simulink library "lib_wheel2"  (Simulink 4.1.1)
values from neighbouring files (symbols this model uses):
  logFlag = 1    [advSACompMaskInit.m]    (also in advSACompMaskInitR13.m)
undefined symbols (not defined in the file or in its folder): lib_help, NOTES, veh_air_density, veh_CD, veh_cg_height, veh_FA, veh_front_wt_frac, veh_gravity, veh_roadwheel_radius, veh_rr_a, veh_rr_alpha, veh_rr_b, veh_rr_beta, veh_rr_c, veh_wheelbase, wh_1st_rrc, wh_2nd_rrc, wh_axle_loss_mass, wh_axle_loss_trq, wh_fa_dl_brake_frac, wh_fa_dl_brake_mph, wh_fa_fric_brake_frac, wh_fa_fric_brake_mph, wh_front_active_bool, wh_inertia, wh_max_front_brake_force, wh_max_rear_brake_force, wh_pressure, wh_radius, wh_rear_active_bool, wh_slip, wh_slip_force_coeff
libraries: lib_wheel2 x61, lib_vehicle x2, lib_etc x2, lib_controls x2, lib_wheel x1
(part 7 of 14)

== system lib_wheel2/Submodels/front and rear brake controller (achievable)/braking force supplied by front friction brakes (N)/Block NOTES ==
  note: The variable "wh_max_front_fric_brake_force_N" must be assigned a positive value.
  note: If all braking was intended to be done by the drivetrain, the front friction brakes will do 60% of the braking.
  note: where the denominator can also be expressed as [1 - front_axle_drivetrain_brake_fraction(vehicle speed)].
  note: [front_axle_friction_brake_fraction(vehicle speed)]
      | ------------------------------------------------------------------------------
      | [front_axle_friction_brake_fraction(vehicle speed) + rear_axle_friction_brake_fraction(vehicle speed)]
  note: If additional braking force is required to meet the specified deceleration, input #1 will be negative.
      | The fraction of the additional req'd braking force made up by the front-axle friction brakes is given by:

== system lib_wheel2/Submodels/traction control 2 axle/apply tire traction limit to req'd speed (m/s)/Block NOTES ==
  note: This block limits the requested speed by the maximum and minimum attainable given the maximum traction of the tires.
      | That is, acceleration and braking maneuvers are limited to the point of imminent skidding.
  note: The above equations are derived by solving F_maxaccel=mass*a_max for the maximum or minimum speed at the end of the time step,
      | given that F_maxaccel depends on the weight borne by the front tires which in turn depends on the vehicle's acceleration rate.
  note: Front-wheel drive is assumed, and weight transfer due to acceleration is included in the calculation of maximum tractive force.

== system lib_wheel2/Submodels/traction control 2 axle/apply tire traction limit to req'd speed (m/s)/max speed at END of time step given tire traction limit (m/s) ==
  in_1 : Inport  Port=1  LatchInput=off
  in_2 : Inport  Port=2  LatchInput=off
  Fcn : Fcn  Expr=1/u
  Product : Product  Inputs=2  Multiplication=Element-wise(.*)  SaturateOnIntegerOverflow=on
  out_1 : Outport  Port=1  InitialOutput=0
  wires:
  in_1/1 -> Product/1
  Fcn/1 -> Product/2
  Product/1 -> out_1/1
  in_2/1 -> Fcn/1

== system lib_wheel2/Submodels/traction control 2 axle/apply tire traction limit to req'd speed (m/s)/min speed at END of time step given tire traction limit (m/s) ==
  in_1 : Inport  Port=1  LatchInput=off
  in_2 : Inport  Port=2  LatchInput=off
  Fcn : Fcn  Expr=1/u
  Product : Product  Inputs=2  Multiplication=Element-wise(.*)  SaturateOnIntegerOverflow=on
  out_1 : Outport  Port=1  InitialOutput=0
  wires:
  in_2/1 -> Fcn/1
  Product/1 -> out_1/1
  Fcn/1 -> Product/2
  in_1/1 -> Product/1

== system lib_wheel2/Submodels/traction control 2 axle/apply tire traction limit to req'd speed (m/s)/rear slip terms ==
  initial speed : Inport  Port=1  LatchInput=off
  1/dt : Inport  Port=2  LatchInput=off
  sin(theta) : Inport  Port=3  LatchInput=off
  Constant12 : Constant  Value=max(wh_slip_force_coeff)*(-1*veh_cg_height)/veh_wheelbase
  Constant8 : Constant  Value=veh_gravity
  Product13 : Product  Inputs=3  Multiplication=Element-wise(.*)  SaturateOnIntegerOverflow=on
  Product14 : Product  Inputs=4  Multiplication=Element-wise(.*)  SaturateOnIntegerOverflow=on
  current veh mass : lib_wheel2/Submodels/current veh mass
      settings: RTWFcnNameOpts=Auto  RTWFileNameOpts=Auto
  Out1 : Outport  Port=1
  Out2 : Outport  Port=2
  wires:
  sin(theta)/1 -> Product13/3
  Product13/1 -> Out2/1
  1/dt/1 -> Product14/3
  Product14/1 -> Out1/1
  initial speed/1 -> Product14/2
  current veh mass/1 -> Product14/4
  Constant8/1 -> Product13/2
  Constant12/1 -> Product13/1, Product14/1

== system lib_wheel2/Submodels/traction control 2 axle/enforce max.  front axle tractive force  due to slip (N)/Block NOTES ==
  note: No more force will be requested of the drivetrain than can be transmitted by the front tires.
      | This transmittable force is computed taking into account the slip characteristics of the tires
      | and the variable, acceleration-dependent weight borne by the front axle.

== system lib_wheel2/Submodels/traction control 2 axle/enforce max.  front axle tractive force  due to slip (N)/front ==
  In1 : Inport  Port=1  LatchInput=off
  In2 : Inport  Port=2  LatchInput=off
  Clock : Clock
      settings: DisplayTime=off  Decimation=10
  Constant : Constant  Orientation=left  Value=veh_cg_height/veh_wheelbase
  Constant1 : Constant  Value=veh_gravity*veh_front_wt_frac
  Gain1 : Gain  Gain=2  Multiplication=Element-wise(K.*u)  SaturateOnIntegerOverflow=on
  Gain2 : Gain  Gain=veh_gravity  Multiplication=Element-wise(K.*u)  SaturateOnIntegerOverflow=on
  Memory1 : Memory  X0=-0.1  InheritSampleTime=off
      settings: RTWStateStorageClass=Auto
  Product : Product  Inputs=*/  Multiplication=Element-wise(.*)  SaturateOnIntegerOverflow=on
  Product1 : Product  Inputs=3  Multiplication=Element-wise(.*)  SaturateOnIntegerOverflow=on
  Product3 : Product  Inputs=3  Multiplication=Element-wise(.*)  SaturateOnIntegerOverflow=on
  Sum : Sum  Inputs=+-  SaturateOnIntegerOverflow=on
  Sum1 : Sum  Inputs=+-  SaturateOnIntegerOverflow=on
  Sum2 : Sum  Inputs=++  SaturateOnIntegerOverflow=on
  Trig Fn : Trigonometry  Operator=atan  OutputSignalType=auto
  Trig Fn1 : Trigonometry  Operator=sin  OutputSignalType=auto
  Trig Fn2 : Trigonometry  Operator=cos  OutputSignalType=auto
  current veh mass2 : lib_wheel2/Submodels/current veh mass
      settings: RTWFcnNameOpts=Auto  RTWFileNameOpts=Auto
  weight on front axle (N)1 : Sum  Inputs=-+  SaturateOnIntegerOverflow=on
  Out1 : Outport  Port=1
  wires:
  weight on front axle (N)1/1 -> Out1/1
  In2/1 -> Sum/2
  In1/1 -> Sum/1
  current veh mass2/1 -> Product3/1, Product1/3
  Trig Fn2/1 -> Product3/2
  Constant1/1 -> Product3/3
  Product3/1 -> weight on front axle (N)1/2
  Trig Fn/1 -> Trig Fn2/1, Trig Fn1/1
  Gain2/1 -> Sum2/2
  Trig Fn1/1 -> Gain2/1
  [grade] -> Trig Fn/1
  Sum2/1 -> Product1/2
  Gain1/1 -> Sum2/1
  Product/1 -> Gain1/1
  Sum1/1 -> Product/2
  Memory1/1 -> Sum1/2
  Clock/1 -> Memory1/1, Sum1/1
  Sum/1 -> Product/1
  Constant/1 -> Product1/1
  Product1/1 -> weight on front axle (N)1/1

== system lib_wheel2/Submodels/traction control 2 axle/enforce max.  front axle tractive force  due to slip (N)/rear ==
  In1 : Inport  Port=1  LatchInput=off
  In2 : Inport  Port=2  LatchInput=off
  Clock : Clock
      settings: DisplayTime=off  Decimation=10
  Constant : Constant  Orientation=left  Value=(-1*veh_cg_height)/veh_wheelbase
  Constant1 : Constant  Value=veh_gravity*(1-veh_front_wt_frac)
  Gain1 : Gain  Gain=2  Multiplication=Element-wise(K.*u)  SaturateOnIntegerOverflow=on
  Gain2 : Gain  Gain=veh_gravity  Multiplication=Element-wise(K.*u)  SaturateOnIntegerOverflow=on
  Memory1 : Memory  X0=-0.1  InheritSampleTime=off
      settings: RTWStateStorageClass=Auto
  Product : Product  Inputs=*/  Multiplication=Element-wise(.*)  SaturateOnIntegerOverflow=on
  Product1 : Product  Inputs=3  Multiplication=Element-wise(.*)  SaturateOnIntegerOverflow=on
  Product3 : Product  Inputs=3  Multiplication=Element-wise(.*)  SaturateOnIntegerOverflow=on
  Sum : Sum  Inputs=+-  SaturateOnIntegerOverflow=on
  Sum1 : Sum  Inputs=+-  SaturateOnIntegerOverflow=on
  Sum2 : Sum  Inputs=++  SaturateOnIntegerOverflow=on
  Trig Fn : Trigonometry  Operator=atan  OutputSignalType=auto
  Trig Fn1 : Trigonometry  Operator=sin  OutputSignalType=auto
  Trig Fn2 : Trigonometry  Operator=cos  OutputSignalType=auto
  current veh mass2 : lib_wheel2/Submodels/current veh mass
      settings: RTWFcnNameOpts=Auto  RTWFileNameOpts=Auto
  weight on rear axle (N) : Sum  Inputs=-+  SaturateOnIntegerOverflow=on
  Out1 : Outport  Port=1
  wires:
  weight on rear axle (N)/1 -> Out1/1
  In2/1 -> Sum/2
  In1/1 -> Sum/1
  current veh mass2/1 -> Product3/1, Product1/3
  Trig Fn2/1 -> Product3/2
  Constant1/1 -> Product3/3
  Product3/1 -> weight on rear axle (N)/2
  Trig Fn/1 -> Trig Fn2/1, Trig Fn1/1
  Gain2/1 -> Sum2/2
  Trig Fn1/1 -> Gain2/1
  [grade] -> Trig Fn/1
  Sum2/1 -> Product1/2
  Gain1/1 -> Sum2/1
  Product/1 -> Gain1/1
  Sum1/1 -> Product/2
  Memory1/1 -> Sum1/2
  Clock/1 -> Memory1/1, Sum1/1
  Sum/1 -> Product/1
  Constant/1 -> Product1/1
  Product1/1 -> weight on rear axle (N)/1

== system lib_wheel2/Submodels/traction control J2452 2 axle/apply tire traction limit to req'd speed (m/s)/Block NOTES ==
  note: This block limits the requested speed by the maximum and minimum attainable given the maximum traction of the tires.
      | That is, acceleration and braking maneuvers are limited to the point of imminent skidding.
  note: The above equations are derived by solving F_maxaccel=mass*a_max for the maximum or minimum speed at the end of the time step,
      | given that F_maxaccel depends on the weight borne by the front tires which in turn depends on the vehicle's acceleration rate.
  note: Front-wheel drive is assumed, and weight transfer due to acceleration is included in the calculation of maximum tractive force.
      |
      | SAE J2452 rolling resistance model is included.
      |
      | Rolling resistance coefficients veh_rr_a and veh_rr_b have units of N/km/h and N/(km/h)^2 respectively.
      | Each is converted to N/m/s and N/(m/s)^2 with the gain blocks before it is input into the final traction equation.
      |
      | Veh_rr_a, veh_rr_b, and veh_rr_c must always be adjusted for roadwheel curvature before use.

== system lib_wheel2/Submodels/traction control J2452 2 axle/apply tire traction limit to req'd speed (m/s)/Subsystem ==
  Constant16 : Constant  Value=(-1*veh_cg_height/veh_wheelbase)
  Constant17 : Constant  Value=wh_radius
  Constant18 : Constant  Value=(1-veh_front_wt_frac)
  Constant19 : Constant  Value=0
  Error Check1 : MinMax  Function=max  Inputs=2
  Memory2 : Memory  Orientation=down  X0=-0.1  InheritSampleTime=off
      settings: RTWStateStorageClass=Auto
  Product10 : Product  Inputs=3  Multiplication=Element-wise(.*)  SaturateOnIntegerOverflow=on
  Product11 : Product  Inputs=2  Multiplication=Element-wise(.*)  SaturateOnIntegerOverflow=on
  Product12 : Product  Inputs=2  Multiplication=Element-wise(.*)  SaturateOnIntegerOverflow=on
  Product13 : Product  Inputs=2  Multiplication=Element-wise(.*)  SaturateOnIntegerOverflow=on
  Sum2 : Sum  Inputs=+-  SaturateOnIntegerOverflow=on
  Sum3 : Sum  Inputs=+-  SaturateOnIntegerOverflow=on
  Sum6 : Sum  Inputs=-+  SaturateOnIntegerOverflow=on
  Trig Fn7 : Trigonometry  Operator=atan  OutputSignalType=auto
  Trig Fn8 : Trigonometry  Operator=cos  OutputSignalType=auto
  current veh mass2 : lib_wheel2/Submodels/current veh mass
      settings: RTWFcnNameOpts=Auto  RTWFileNameOpts=Auto
  Out1 : Outport  Port=1
  Out2 : Outport  Port=2
  wires:
  Error Check1/1 -> Sum6/1, Out1/1  "Nf"
  Constant19/1 -> Error Check1/2
  Sum2/1 -> Error Check1/1  "Nf"
  Product13/1 -> Sum6/2  "W"
  Memory2/1 -> Product11/1
  [wh_trq_a] -> Memory2/1
  current veh mass2/1 -> Product13/2, Product10/3
  Constant18/1 -> Product10/2
  Trig Fn8/1 -> Product13/1, Product10/1
  Trig Fn7/1 -> Trig Fn8/1
  [grade] -> Trig Fn7/1
  Product10/1 -> Sum2/1
  Constant17/1 -> Product11/2
  Product11/1 -> Sum3/1
  [Fr_out] -> Sum3/2
  Sum3/1 -> Product12/1
  Constant16/1 -> Product12/2
  Product12/1 -> Sum2/2
  Sum6/1 -> Out2/1  "Nr=W-Nf"

== system lib_wheel2/Submodels/traction control J2452 2 axle/apply tire traction limit to req'd speed (m/s)/Subsystem1 ==
  Constant15 : Constant  Value=max(wh_slip_force_coeff)*veh_gravity*(1-veh_front_wt_frac)
  Product8 : Product  Inputs=3  Multiplication=Element-wise(.*)  SaturateOnIntegerOverflow=on
  Trig Fn5 : Trigonometry  Operator=atan  OutputSignalType=auto
  Trig Fn6 : Trigonometry  Operator=cos  OutputSignalType=auto
  current veh mass2 : lib_wheel2/Submodels/current veh mass
      settings: RTWFcnNameOpts=Auto  RTWFileNameOpts=Auto
  Out1 : Outport  Port=1
  wires:
  Trig Fn6/1 -> Product8/2
  current veh mass2/1 -> Product8/3
  Constant15/1 -> Product8/1
  Trig Fn5/1 -> Trig Fn6/1
  [grade] -> Trig Fn5/1
  Product8/1 -> Out1/1  "Ftract"

== system lib_wheel2/development/wheel and axle  front/rear <wh>/wheel & axle model & interface/signal annotator ==
  In1 : Inport  Port=1  LatchInput=off
  Demux : Demux  Outputs=2  BusSelectionMode=off
  Mux : Mux  Inputs=2
  Out1 : Outport  Port=1
  wires:
  In1/1 -> Demux/1
  Demux/1 -> Mux/1  "F_traction_r"
  Demux/2 -> Mux/2  "veh_speed_r"
  Mux/1 -> Out1/1
